simulink model "pO"  (Simulink 7.5)
settings: Solver=ode45  StartTime=0.0  StopTime=10.0  RelTol=1e-3
libraries: simulink x7
settings Model: Creator=dell  LastModifiedBy=dell

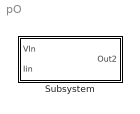
== system pO ==
  Subsystem : Subsystem

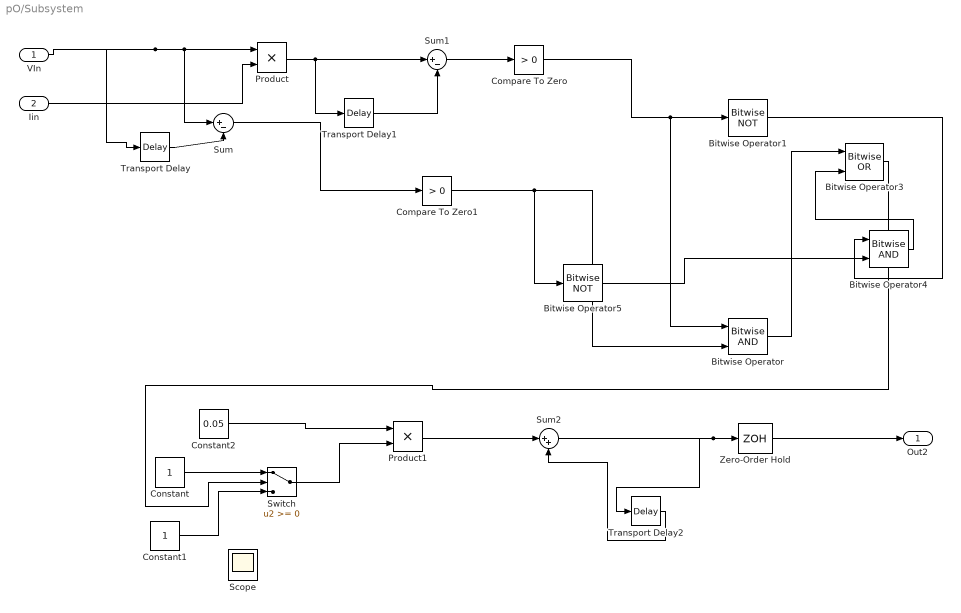
== system pO/Subsystem ==
  VIn : Inport  OutDataType=fixdt(1, 16)  OutScaling=2^0
  Iin : Inport  Port=2  OutDataType=fixdt(1, 16)  OutScaling=2^0
  Bitwise Operator : simulink/Logic and Bit Operations/Bitwise Operator  logicop=AND  UseBitMask=off  NumInputPorts=2  BitMask=bin2dec('11011001')  BitMaskRealWorld=Real World Value
  Bitwise Operator1 : simulink/Logic and Bit Operations/Bitwise Operator  logicop=NOT  UseBitMask=off  BitMask=bin2dec('11011001')  BitMaskRealWorld=Real World Value
  Bitwise Operator3 : simulink/Logic and Bit Operations/Bitwise Operator  logicop=OR  UseBitMask=off  NumInputPorts=2  BitMask=bin2dec('11011001')  BitMaskRealWorld=Real World Value
  Bitwise Operator4 : simulink/Logic and Bit Operations/Bitwise Operator  logicop=AND  UseBitMask=off  NumInputPorts=2  BitMask=bin2dec('11011001')  BitMaskRealWorld=Real World Value
  Bitwise Operator5 : simulink/Logic and Bit Operations/Bitwise Operator  logicop=NOT  UseBitMask=off  BitMask=bin2dec('11011001')  BitMaskRealWorld=Real World Value
  Compare To Zero : simulink/Logic and Bit Operations/Compare To Zero  SystemSampleTime=-1  relop=>  LogicOutDataTypeMode=uint8
  Compare To Zero1 : simulink/Logic and Bit Operations/Compare To Zero  SystemSampleTime=-1  relop=>  LogicOutDataTypeMode=uint8
  Constant : Constant  OutDataType=fixdt(1, 16)  OutScaling=2^0
  Constant1 : Constant  OutDataType=fixdt(1, 16)  OutScaling=2^0
  Constant2 : Constant  Value=0.05  OutDataType=fixdt(1, 16)  OutScaling=2^0
  Product : Product  OutDataType=fixdt(1, 16)  OutScaling=2^0  RndMeth=Zero
  Product1 : Product  OutDataType=fixdt(1, 16)  OutScaling=2^0  RndMeth=Zero
  Scope : Scope
  Sum : Sum  Inputs=|+-  OutDataType=fixdt(1, 16)  OutScaling=2^0
  Sum1 : Sum  Inputs=|+-  OutDataType=fixdt(1, 16)  OutScaling=2^0
  Sum2 : Sum  Inputs=|++  OutDataType=fixdt(1, 16)  OutScaling=2^0
  Switch : Switch  OutDataType=fixdt(1, 16)  OutScaling=2^0
  Transport Delay : TransportDelay
  Transport Delay1 : TransportDelay
  Transport Delay2 : TransportDelay
  Zero-Order Hold : ZeroOrderHold
  Out2 : Outport  OutDataType=fixdt(1, 16)  OutScaling=2^0
  wires:
  VIn/1 -> Transport Delay/1, Product/1, Sum/1
  Transport Delay/1 -> Sum/2
  Iin/1 -> Product/2
  Product/1 -> Sum1/1, Transport Delay1/1
  Transport Delay1/1 -> Sum1/2
  Sum1/1 -> Compare To Zero/1
  Compare To Zero/1 -> Bitwise Operator1/1, Bitwise Operator/1
  Bitwise Operator/1 -> Bitwise Operator3/1
  Sum/1 -> Compare To Zero1/1
  Compare To Zero1/1 -> Bitwise Operator/2, Bitwise Operator5/1
  Bitwise Operator1/1 -> Bitwise Operator4/1
  Bitwise Operator4/1 -> Bitwise Operator3/2
  Bitwise Operator5/1 -> Bitwise Operator4/2
  Constant/1 -> Switch/1
  Constant1/1 -> Switch/3
  Bitwise Operator3/1 -> Switch/2
  Constant2/1 -> Product1/1
  Switch/1 -> Product1/2
  Product1/1 -> Sum2/1
  Sum2/1 -> Zero-Order Hold/1, Transport Delay2/1
  Transport Delay2/1 -> Sum2/2
  Zero-Order Hold/1 -> Out2/1
